simulink model "AJAC_Simulation"  (R2024b)
settings: Solver=FixedStepAuto  StartTime=0.0  StopTime=1  FixedStep=0.000025  RelTol=1e-7  EnableMultiTasking=on
InitFcn:
  | Ld=5.25e-3;
  | Lq=12e-3;
  | R=0.958;
  | f=0.1827;
model workspace (MAT data in the model file):
  f : Simulink.Signal (value not decoded)
libraries: slpidlib x2, mcbplantlib x1, simulink x1, spsPermanentMagnetSynchronousMachineLib x1, autolibpmsmexterior x1, spspowerguiLib x1
(part 2 of 2)

== matlab function AJAC_Simulation/Only_Stable_Motor_VK ==
  settings: updateMethod=DISCRETE  sampleTime=0.001
  data: res_uq output; res_ud output; we_k_1 input; we_k_2 input; iq_k_1 input; uq_k_1 input; ud_k_1 input; L_s input; R_s input; f data_store_memory; iq_lb output; iq_ub output; phi_m input; V_bound input; out_iq_k_1 output; out_we_k_1 output; epsilon output; iq_out output; last_delta_uq input; iq_ref input; tau_ff input
function [res_uq, res_ud,iq_lb, iq_ub, out_iq_k_1, out_we_k_1, epsilon, iq_out] = fcn(we_k_1, we_k_2 , iq_k_1, uq_k_1, ud_k_1,L_s, R_s, phi_m, V_bound, last_delta_uq,iq_ref, tau_ff)

delta_t = 0.001; %second
Inertial_Rotor = 0.0003;
Npp = 21;
iq_max = 30;
delta_uq = 0;
delta_ud = 0;
delta_uq_gain = 1.0;
steps = 100;

% try integral, integral works.
filter = 0.1;
delta_uq = (uq_k_1 - (R_s * iq_k_1 + we_k_1* phi_m)) * filter + (1-filter) * last_delta_uq;
% delta_uq = uq_k_1 - (R_s * iq_k_1 + we_k_1* phi_m);
delta_ud = ud_k_1 - (-we_k_2 * L_s * iq_k_1);

m = R_s + (3*phi_m*phi_m*Npp * steps * delta_t)/(2*Inertial_Rotor);
n = (we_k_1 - (tau_ff * delta_t * steps)/(Inertial_Rotor))*phi_m + delta_uq;
p = -we_k_1* L_s;

estimated_vel = we_k_1 + (1.5*phi_m*Npp * iq_k_1) * steps * delta_t;

epsilon = 2*m*n*p*delta_ud + m*m*V_bound*V_bound + p*p*V_bound*V_bound - m*m*delta_ud*delta_ud - p*p*n*n;
epsilon_judgement_1 = sqrt(m*m+p*p)*V_bound - (m*delta_ud - p*n);
epsilon_judgement_2 = sqrt(m*m+p*p)*V_bound + m*delta_ud - p *n;
% ep_fake = (V_bound*sqrt(m*m+p*p))^2-(m*delta_ud - p*n)^2;
judge_1 = epsilon_judgement_1;
judge_2 = epsilon_judgement_2;

iq_lb_temp = 0;
iq_ub_temp = 0;
out_iq_k_1 = iq_k_1;
out_we_k_1 = we_k_1;

if epsilon >= 0
    iq_lb_temp = (-m*n - p*delta_ud - sqrt(epsilon)) / (m * m + p * p);
    iq_ub_temp = (-m*n - p* delta_ud +  sqrt(epsilon)) / (m * m + p * p);
else
    
end
%%

iq_lb = iq_lb_temp;
if(iq_lb > 0)
    iq_lb = 0;
end
iq_ub = iq_ub_temp;
if(iq_ub < 0)
    iq_ub = 0;
end

% Del's paper only consider the decelerate.
% if (iq_ref * we_k_1) > 0 && (iq_ref > 0)
%     % the same direction
%     iq_lb = -25;
% end

% if (iq_ref * we_k_1) > 0 && (iq_ref < 0)
%     % the same direction
%     iq_ub = 25;
% end

res_uq = delta_uq;
res_ud = delta_ud;
iq_out = max([iq_lb,min([iq_ref, iq_ub])]);

== matlab function AJAC_Simulation/pos_vel_vk ==
  settings: updateMethod=DISCRETE  sampleTime=0.001
  data: ddq_max input; q_k_1 input; dq_k_1 input; delta_t input; q_min input; q_max input; ddq_lb output; ddq_ub output; dq_max input; iq_ref input; N_step input; phi_m input; inertia input; iq_ref_out output; ddq_ref_clipped output; ddq_ref output
function [ddq_lb, ddq_ub, iq_ref_out, ddq_ref_clipped, ddq_ref]  = fcn(ddq_max, q_k_1, dq_k_1, delta_t, q_min, q_max, dq_max, iq_ref, N_step, phi_m, inertia)

ddq_lb_pos = 0;
ddq_ub_pos = 0;
ddq_lb_vel = 0;
ddq_ub_vel = 0;
Np = 21;

%% acc from the pos Limits
ddq_M1 = -dq_k_1 / (N_step *delta_t);
ddq_M2 = -dq_k_1*dq_k_1 /(2*(q_max-q_k_1));
ddq_M3 = 2*(q_max - q_k_1 - N_step * delta_t* dq_k_1)/(N_step * delta_t * delta_t);
ddq_m2 = dq_k_1 * dq_k_1 / (2 * (q_k_1 - q_min));
ddq_m3 = 2 * (q_min - q_k_1 - N_step * delta_t * dq_k_1)/(N_step * delta_t * delta_t);

if dq_k_1 >= 0 
    ddq_lb_pos = ddq_m3;
    if ddq_M3 > ddq_M1
        ddq_ub_pos = ddq_M3;
    else
        ddq_ub_pos = min([ddq_M1, ddq_M2]);
    end
else
    ddq_ub_pos = ddq_M3;
    if ddq_m3 < ddq_M1
        ddq_lb_pos = ddq_m3;
    else
        ddq_lb_pos = max([ddq_M1, ddq_m2]);
    end
end

%% acc bounds from viability
a = N_step * N_step *delta_t * delta_t;
b = N_step*delta_t *(2*dq_k_1 + ddq_max  * N_step*delta_t);
c = dq_k_1 * dq_k_1 - 2 * ddq_max * (q_max - q_k_1 - N_step*delta_t*dq_k_1);
ddq_1 = -dq_k_1 / (N_step*delta_t);
epsilon = b*b - 4*a*c;
if epsilon >= 0
    ddq_ub_vel = max([ddq_1, (-b+sqrt(epsilon))/(2*a)]);
else
    ddq_ub_vel = ddq_1;
end
% negative speed
b = 2*N_step*delta_t*dq_k_1 - ddq_max * N_step*N_step*delta_t * delta_t;
c = dq_k_1*dq_k_1 - 2 * ddq_max * (q_k_1 + N_step*delta_t*dq_k_1 - q_min);
epsilon = b*b - 4*a*c;
if epsilon >=0
    ddq_lb_vel = min([ddq_1,(-b-sqrt(epsilon))/(2*a)]);
else
    ddq_lb_vel = ddq_1;
end

%%
ddq_ub_1 = ddq_max;
ddq_ub_2 = ddq_ub_pos;
ddq_ub_3 = ddq_ub_vel;
ddq_ub_4 = (dq_max - dq_k_1)/(N_step*delta_t);

ddq_lb_1 = -ddq_max;
ddq_lb_2 = ddq_lb_pos;
ddq_lb_3 = ddq_lb_vel;
ddq_lb_4 = (-dq_max - dq_k_1)/(N_step*delta_t);

% return the final
ddq_lb = max([ddq_lb_1, ddq_lb_2, ddq_lb_3, ddq_lb_4]);
ddq_ub = min([ddq_ub_1, ddq_ub_2, ddq_ub_3, ddq_ub_4]);

%% output the acc:
% ddq_ref = 1000 * (q_ref - q_k_1) - 10 * dq_k_1;
ddq_ref = iq_ref * 1.5 * phi_m * Np / inertia;  % 0.13 here is for kt.
ddq_ref_clipped = max([min([ddq_ref, ddq_ub]), ddq_lb]);
% transform ddq to iq
iq_ref_out = ddq_ref_clipped * 2*inertia / (3*Np*phi_m);

== matlab function AJAC_Simulation/Encoder ==
  settings: updateMethod=DISCRETE  sampleTime=0.000025
  data: loop_count input; pos_global output; loop_count_out output; pos_2pi input; pos_2pi_out output; last_pos_2pi input
function [pos_global, loop_count_out, pos_2pi_out] = fcn(loop_count, pos_2pi, last_pos_2pi)
pos_2pi_out = pos_2pi;

if(pos_2pi - last_pos_2pi > pi)
    loop_count = loop_count - 1;
elseif(pos_2pi - last_pos_2pi < -pi)
    loop_count = loop_count + 1;
end

pos_global = loop_count*2*pi + pos_2pi;
loop_count_out = loop_count;
